simulink model "clik_z_inverse"  (Simulink 10.2)
settings: Solver=VariableStepAuto  StartTime=0.0  StopTime=4  RelTol=1e-3
undefined symbols (not defined in the file or in its folder): DiscIntNeverNeededParam, q0, Tc
settings Model: Creator=Megha  LastModifiedBy=Megha
settings DataIOCC: SaveFormat=Dataset  SignalLoggingSaveFormat=Dataset  ReturnWorkspaceOutputs=on
settings OptimizationCC: LifeSpan=auto
settings DebuggingCC: UnderspecifiedInitializationDetection=Simplified  MergeDetectMultiDrivingBlocksExec=error  FcnCallInpInsideContextMsg=error  SFUnexpectedBacktrackingDiag=error  SFNoUnconditionalDefaultTransitionDiag=error  SFExecutionAtInitializationDiag=warning  ArithmeticOperatorsInVariantConditions=error
settings HardwareCC: ProdBitPerPointer=64  ProdBitPerSizeT=64  ProdBitPerPtrDiffT=64  ProdLargestAtomicFloat=Float  ProdIntDivRoundTo=Zero  ProdEndianess=LittleEndian  ProdWordSize=64  ProdHWDeviceType=Intel->x86-64 (Windows64)
settings ModelReferenceCC: PropagateSignalLabelsOutOfModel=on
settings SFSimCC: SimUseLocalCustomCode=on  CustomCodeUndefinedFunction=FilterOut
settings RTWCC: RTWUseLocalCustomCode=on
settings CodeAppCC: StateflowObjectComments=off
settings GRTTargetCC: TargetLangStandard=C99 (ISO)  CombineOutputUpdateFcns=on  GRTInterface=off
settings ConfigComp: CovMetricSettings=dwe  CovSaveCumulativeToWorkspaceVar=off  CovSaveSingleToWorkspaceVar=off  CovExternalEMLEnable=on

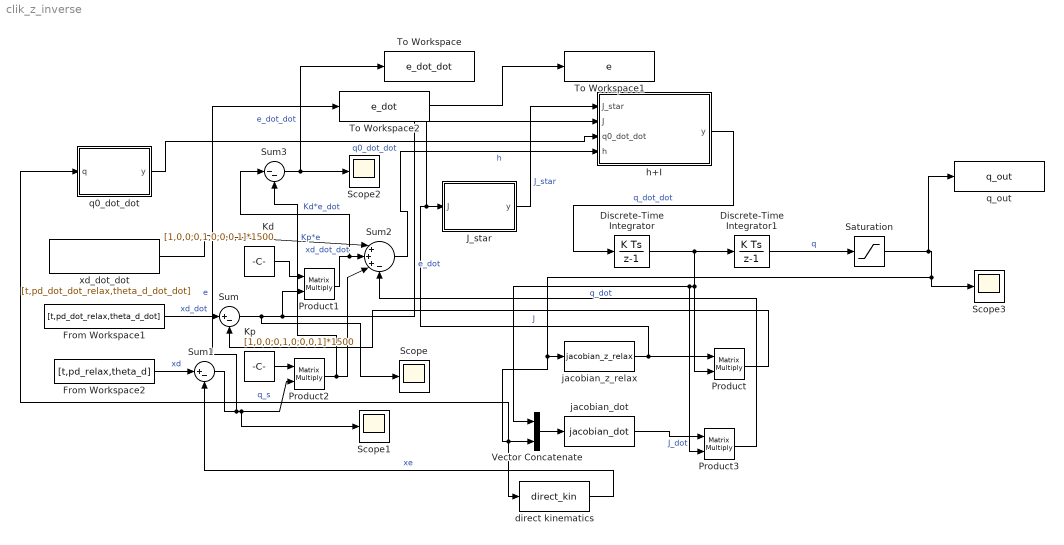
== system clik_z_inverse ==
  Discrete-Time Integrator : DiscreteIntegrator  SampleTime=Tc  ICPrevOutput=DiscIntNeverNeededParam  ICPrevScaledInput=DiscIntNeverNeededParam
  Discrete-Time Integrator1 : DiscreteIntegrator  InitialCondition=q0  SampleTime=Tc  ICPrevOutput=DiscIntNeverNeededParam  ICPrevScaledInput=DiscIntNeverNeededParam
  From Workspace1 : FromWorkspace  VariableName=[t,pd_dot_relax,theta_d_dot]
  From Workspace2 : FromWorkspace  VariableName=[t,pd_relax,theta_d]
  J_star : MATLAB Function  TreatAsAtomicUnit=on
  Kd : Constant  Value=[1,0,0;0,1,0;0,0,1]*1500  VectorParams1D=off
  Kp : Constant  Value=[1,0,0;0,1,0;0,0,1]*1500  VectorParams1D=off
  Product{,1..3} (4 alike) : Product  Multiplication=Matrix(*)
  Saturation : Saturate  UpperLimit=[pi/2 , pi/4 , 1 , 2*pi]  LowerLimit="[-pi/2 , -pi/2, 0.25  -2*pi]"
  Scope{,1..3} (4 alike) : Scope
  Sum : Sum  Inputs=|+-
  Sum1 : Sum  Inputs=|+-
  Sum2 : Sum  Inputs=|+++-
  Sum3 : Sum  Inputs=|--
  To Workspace : ToWorkspace  VariableName=e_dot_dot  SampleTime=-1
  To Workspace1 : ToWorkspace  VariableName=e  SampleTime=-1
  To Workspace2 : ToWorkspace  VariableName=e_dot  SampleTime=-1
  Vector Concatenate : Concatenate
  direct kinematics : MATLABFcn  MATLABFcn=direct_kin  Output1D=off
  h+I : MATLAB Function  TreatAsAtomicUnit=on
  jacobian_dot : MATLABFcn  MATLABFcn=jacobian_dot  Output1D=off
  jacobian_z_relax : MATLABFcn  MATLABFcn=jacobian_z_relax  Output1D=off
  q0_dot_dot : MATLAB Function  TreatAsAtomicUnit=on
  q_out : ToWorkspace  VariableName=q_out  SampleTime=Tc
  xd_dot_dot : FromWorkspace  VariableName=[t,pd_dot_dot_relax,theta_d_dot_dot]
  wires:
  From Workspace1/1 -> Sum/1  "xd_dot"
  From Workspace2/1 -> Sum1/1  "xd"
  xd_dot_dot/1 -> Sum2/1  "xd_dot_dot"
  Discrete-Time Integrator/1 -> Product3/2, Vector Concatenate/1, Product/2, Discrete-Time Integrator1/1  "q_dot"
  jacobian_z_relax/1 -> h+I/2(J), J_star/1(J), Product/1  "J"
  Product/1 -> Sum/2
  Sum1/1 -> To Workspace2/1, Scope1/1, Product2/2  "e"
  direct kinematics/1 -> Sum1/2  "xe"
  Kd/1 -> Product1/1
  Sum/1 -> To Workspace1/1, Product1/2, Scope/1  "e_dot"
  Product1/1 -> Sum3/1, Sum2/2  "Kd*e_dot"
  Kp/1 -> Product2/1
  Product2/1 -> Sum3/2, Sum2/3  "Kp*e"
  Vector Concatenate/1 -> jacobian_dot/1
  Sum2/1 -> h+I/4(h)  "h"
  q0_dot_dot/1(y) -> h+I/3(q0_dot_dot)  "q0_dot_dot"
  J_star/1(y) -> h+I/1(J_star)  "J_star"
  h+I/1(y) -> Discrete-Time Integrator/1  "q_dot_dot"
  Saturation/1 -> q_out/1, q0_dot_dot/1(q), direct kinematics/1, Vector Concatenate/2, jacobian_z_relax/1, Scope3/1  "q_s"
  Discrete-Time Integrator1/1 -> Saturation/1  "q"
  jacobian_dot/1 -> Product3/1  "J_dot"
  Product3/1 -> Sum2/4
  Sum3/1 -> To Workspace/1, Scope2/1  "e_dot_dot"

== matlab function J_star ==
  data: J input double; y output double
function y = fcn(J)
J_star = (J.') * inv(J*J.');
y = J_star;

== matlab function h+I ==
  data: J_star input double; y output double; J input double; q0_dot_dot input double; h input double
function y = fcn(J_star,J,q0_dot_dot,h)
l = (eye(4)-(J_star*J))*q0_dot_dot;

q_dot_dot = J_star*(h) + l;
y = q_dot_dot;

== matlab function q0_dot_dot ==
  data: q input double; y output double
function y = fcn(q)
theta_1 = q(1);
theta_2 = q(2);
d3 = q(3);
theta_4 = q(4);
q1 =[2*(cos(theta_1)/2 + (cos(theta_1)*cos(theta_2))/2 - (sin(theta_1)*sin(theta_2))/2)^2 - 2*(sin(theta_1)/2 + (cos(theta_1)*sin(theta_2))/2 + (cos(theta_2)*sin(theta_1))/2)*(sin(theta_1)/2 + (cos(theta_1)*sin(theta_2))/2 + (cos(theta_2)*sin(theta_1))/2 + 7/10) - 2*(cos(theta_1)/2 + (cos(theta_1)*cos(theta_2))/2 - (sin(theta_1)*sin(theta_2))/2)*(cos(theta_1)/2 + (cos(theta_1)*cos(theta_2))/2 - (sin(theta_1)*sin(theta_2))/2 - 2/5) + 2*(sin(theta_1)/2 + (cos(theta_1)*sin(theta_2))/2 + (cos(theta_2)*sin(theta_1))/2)^2];
q2 =[2*((cos(theta_1)*cos(theta_2))/2 - (sin(theta_1)*sin(theta_2))/2)^2 - 2*((cos(theta_1)*sin(theta_2))/2 + (cos(theta_2)*sin(theta_1))/2)*(sin(theta_1)/2 + (cos(theta_1)*sin(theta_2))/2 + (cos(theta_2)*sin(theta_1))/2 + 7/10) - 2*((cos(theta_1)*cos(theta_2))/2 - (sin(theta_1)*sin(theta_2))/2)*(cos(theta_1)/2 + (cos(theta_1)*cos(theta_2))/2 - (sin(theta_1)*sin(theta_2))/2 - 2/5) + 2*((cos(theta_1)*sin(theta_2))/2 + (cos(theta_2)*sin(theta_1))/2)^2];
q3 =[2];
q4 =[0]; 
q0_dot_dot = [q1;q2;q3;q4];
y = q0_dot_dot;
end
